simulink model "ACC_LQR_Gov_STALE"  (R2024a)
settings: Solver=FixedStepAuto  StartTime=0  StopTime=100  FixedStep=.05  RelTol=1e-3
undefined symbols (not defined in the file or in its folder): acc_max, acc_max_tight, Defined, driver_set_speed, Ego, jerk_max, k_I, k_vh, Lane, m, matlabshared, simStepSize, tau_lpf, User, v_dot_max
libraries: roadrunnerscenario x5, drivingscenarioandsensors x1, autolibshared x1
settings Model: PacingRate=10  Creator=darkh  LastModifiedBy=darkh
settings DataIOCC: ReturnWorkspaceOutputsName=sltest_internal_rrSimulationOutputVariable
settings OptimizationCC: ZeroExternalMemoryAtStartup=off  ZeroInternalMemoryAtStartup=off
settings DebuggingCC: AlgebraicLoopMsg=none
settings RTWCC: Description=Generate an RTMaps component embedding the model  SystemTargetFile=rtmaps.tlc  TemplateMakefile=rtmaps_default_tmf  PostCodeGenCommand=rtmaps_post_code_generation(buildInfo)  RetainRTWFile=on  TargetLang=C++  GPUComputeCapability=3.5
settings STFCustomTargetCC: TargetLangStandard=C++11 (ISO)  ModelReferenceCompliant=off  ConcurrentExecutionCompliant=on  CombineOutputUpdateFcns=on  CodeInterfacePackaging=C++ class  CPPClassGenCompliant=on  GRTInterface=off  UseToolchainInfoCompliant=off  SystemTargetFile=rtmaps.tlc
settings GRTTargetCC: TargetLangStandard=C++11 (ISO)  ModelReferenceCompliant=off  ParMdlRefBuildCompliant=off  CompOptLevelCompliant=off  MatFileLogging=off  CodeInterfacePackaging=C++ class  UseToolchainInfoCompliant=off
settings ConfigComp: CovSaveName=sltest_covdata  CovMetricSettings=dcmwe  CovEnableCumulative=off  CovSaveSingleToWorkspaceVar=on  CovSaveOutputData=off

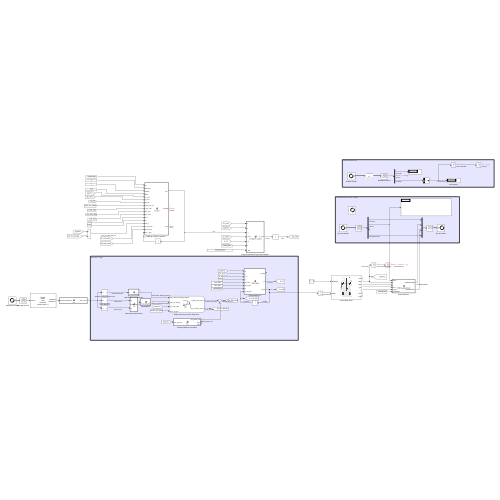
[thumbnail: Simulink's stored preview of the top-level diagram]
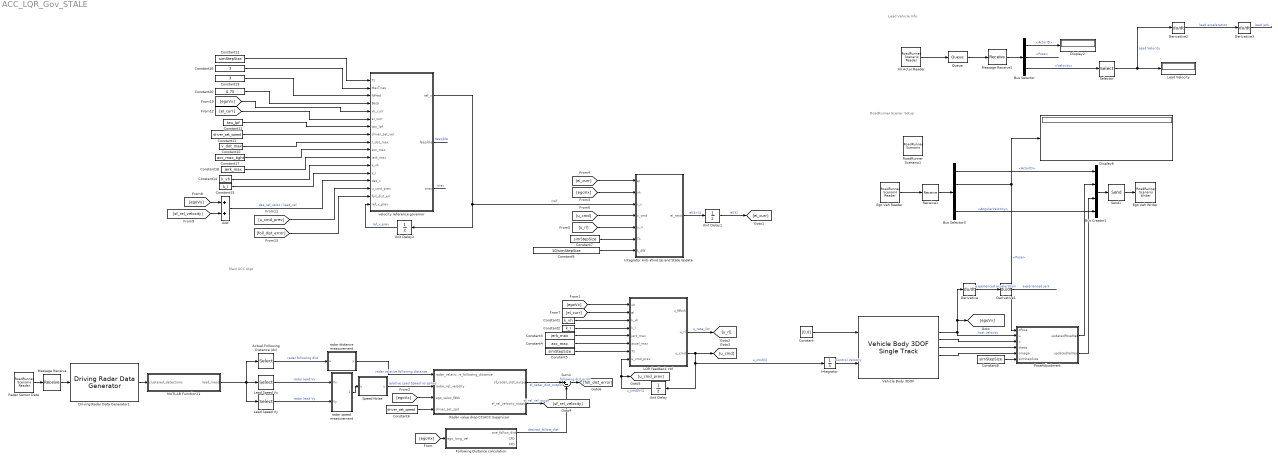
== system ACC_LQR_Gov_STALE ==
  note: RoadRunner Scenar. Setup
  note: Lead Vehicle Info.
  note: Main ACC Algo
  Actual Following Distance (dx) : Selector  InputPortWidth=6  IndexOptions=Index vector (dialog)  Indices=[1]  OutputSizes=1
  Add : Sum
  All Actor Reader : roadrunnerscenario/RoadRunner Scenario Reader  TopicCategory=Actor  ActorCategory=All Types  ActionType=Path Following  EventType=User-Defined  TopicType=Actor Pose  VehicleType=Vehicle Specifications  UserDefinedAction=Action1  UserDefinedEvent=Event1  Filter=None  SensorTopic=Target Poses  LaneBoundaryOutputTopic=Ego-Lane  SensorID=1  SampleTime=simStepSize
  Bus Creator1 : BusCreator  Inputs=4  OutDataTypeStr=Bus: BusActorRuntime  NonVirtualBus=on
      settings: InheritFromInputs=off
  Bus Selector : BusSelector  OutputSignals=ActorID,Pose,Velocity
  Bus Selector3 : BusSelector  OutputSignals=ActorID,Pose,Velocity,AngularVelocity
  Constant : Constant  Value=[0,0]
  Constant1 : Constant  Value=k_vh
  Constant10 : Constant  Value=v_dot_max
  Constant11 : Constant  Value=driver_set_speed
  Constant{5,7..8,12} (4 alike) : Constant  Value=simStepSize
  Constant13 : Constant  Value=tau_lpf
  Constant14 : Constant  Value=k_vh
  Constant15 : Constant  Value=k_I
  Constant16 : Constant  Value=3
  Constant17 : Constant  Value=acc_max_tight
  Constant18 : Constant  Value=jerk_max
  Constant19 : Constant  Value=3
  Constant2 : Constant  Value=k_I
  Constant20 : Constant  Value=0.75
  Constant3 : Constant  Value=jerk_max
  Constant4 : Constant  Value=acc_max
  Constant6 : Constant  Value=driver_set_speed
  Constant9 : Constant  Value=10/simStepSize
  Derivative{,1..3} (4 alike) : Derivative
  Display2 : Display
  Display6 : Display
  Driving Radar Data Generator1 : drivingscenarioandsensors/Driving Radar Data Generator  SensorIndex=1  UpdateRate=20  MountingLocation=[ 3.4, 0, 0.2 ]  MountingAngles=[0 0 0]  HasElevation=off  HasRangeRate=on  HasNoise=off  HasFalseAlarms=off  HasOcclusion=on  MaxNumReportsSource=Property  MaxNumReports=50  TargetReportFormat=Clustered detections  DetectionCoordinates=Body  TrackCoordinates=Body  BusNameSource=Auto  BusName=BusDrivingRadarDataGenerator  AzimuthResolution=4  ElevationResolution=5  RangeResolution=2.5  RangeRateResolution=0.5  AzimuthBiasFraction=0.1  ElevationBiasFraction=0.1  RangeBiasFraction=0.05  RangeRateBiasFraction=0.05  FieldOfView=[ 20, 5 ]  RangeLimits=[ 0, 150 ]  RangeRateLimits=[ -100, 100 ]  DetectionProbability=0.9  FalseAlarmRate=1e-06  ReferenceRange=100  ReferenceRCS=0  CenterFrequency=77e9  FilterInitializationFcn=initcvekf  ConfirmationThreshold=[2 3]  DeletionThreshold=[5 5]  InitialSeedSource=Repeatable  InitialSeed=0  UsedSeed=matlabshared.tracking.internal.SimulinkUtilities.seedManager(gcb)  ProfilesSource=From Scenario Reader block  ProfilesParameters=driving.internal.ActorProfilesRadarParameters  ProfilesExpression=struct('ClassID',0,'Length',4.7,'Width',1.8,'Height',1.4,'OriginOffset',[-1.35 0 0],'RCSPattern',[10 10;10 10],'RCSAzimuthAngles',[-180 180],'RCSElevationAngles',[-90 90])
  Ego Veh Reader : roadrunnerscenario/RoadRunner Scenario Reader  TopicCategory=Actor  ActorCategory=All Types  ActionType=Path Following  EventType=User-Defined  TopicType=Actor Pose  VehicleType=Vehicle Specifications  UserDefinedAction=Action1  UserDefinedEvent=Event1  Filter=Self  SensorTopic=Target Poses  LaneBoundaryOutputTopic=Ego-Lane  SensorID=1  SampleTime=simStepSize
  Ego Veh Writer : roadrunnerscenario/RoadRunner Scenario Writer  TopicCategory=Actor  ActorCategory=All Types  EventType=Action Complete  UserDefinedEvent=Event1  VehicleType=Vehicle Pose  TopicType=Actor Pose
  Following Distance calculation : MATLAB Function  TreatAsAtomicUnit=on
  Integrator : Integrator
  Integrator Anti-Wind Up and State Update : MATLAB Function  TreatAsAtomicUnit=on
  LQR feedback ctrl : MATLAB Function  TreatAsAtomicUnit=on
  Lead Speed Vx : Selector  InputPortWidth=6  IndexOptions=Index vector (dialog)  Indices=4  OutputSizes=1
  Lead Speed Vy : Selector  InputPortWidth=6  IndexOptions=Index vector (dialog)  Indices=5  OutputSizes=1
  Lead Velocity : Display
  MATLAB Function11 : MATLAB Function  TreatAsAtomicUnit=on
  Message Receive : Receive  InputPortMessageModes=m  UseInternalQueue=off
  Message Receive1 : Receive  InputPortMessageModes=m
  PoseAdjustment : MATLAB Function  TreatAsAtomicUnit=on
  Queue : Queue  InputPortMessageModes=m  OutputPortMessageModes=m  OverwriteOldest=on  Capacity=16  QueueType=LIFO
  Radar Sensor Data : roadrunnerscenario/RoadRunner Scenario Reader  TopicCategory=Sensor  ActorCategory=All Types  ActionType=Path Following  EventType=User-Defined  TopicType=Actor Specifications  VehicleType=Vehicle Specifications  UserDefinedAction=Action1  UserDefinedEvent=Event1  Filter=Self  SensorTopic=Target Poses  LaneBoundaryOutputTopic=Ego-Lane  SensorID=1  SampleTime=simStepSize
  Radar value drop CC/ACC Supervisor : Stateflow chart  TreatAsAtomicUnit=on
  Receive1 : Receive  InputPortMessageModes=m  UseInternalQueue=off  QueueOverwriting=on  QueueLength=1  QueueType=LIFO
  RoadRunner Scenario1 : roadrunnerscenario/RoadRunner Scenario  UserDefinedActions={}  UserDefinedEvents={}
  Selector : Selector  InputPortWidth=3  IndexOptions=Index vector (dialog)  Indices=[2]  OutputSizes=1
  Send1 : Send  OutputPortMessageModes=m
  Speed Noise : MATLAB Function  TreatAsAtomicUnit=on
  Sum4 : Sum  Inputs=|+-
  Unit Delay : UnitDelay  SampleTime=-1  HasFrameUpgradeWarning=on
  Unit Delay1 : UnitDelay  SampleTime=-1  HasFrameUpgradeWarning=on
  Unit Delay2 : UnitDelay  SampleTime=-1  HasFrameUpgradeWarning=on
  "Vehicle Body 3DOF " : autolibshared/Vehicle Body 3DOF Single Track  trackMode=Dual  inputMode=External longitudinal velocity  frontSteerMode=on  rearSteerMode=off  windMode=off  muMode=off  extFMode=off  extMMode=off  htchFMode=off  htchMMode=off  extXo=off  extpsio=off  extxdoto=off  extro=off  extYo=off  extTamb=off  extydoto=off  aMode=2  NF=2  NR=2  m=m  a=1.5569  b=1.5371  h=0.18903  dh=1  hh=0.2  X_o=0  xdot_o=0  CalphaMode=off  sigmaMode=on  d=0  hl=0  w=[1.4,1.4]  Cy_f=40000  Cy_r=40000  sigma_f=.1  sigma_r=.1  alpha_f_brk=[-.1 .1]  Cy_f_data=[-9e3 9e3]  alpha_r_brk=[-.1 .1]  Cy_r_data=[-9e3 9e3]  Y_o=0  ydot_o=0  Izz=2066  psi_o=0  r_o=0  Af=2.73  Cd=.30356  Cl=.1  Cpm=.1  beta_w=[0 0.01:0.01:0.3]  Cs=[0 0.01:0.01:0.3]  Cym=[0 1e-6:0.01:0.3]  Pabs=101325  Tair=273  g=9.81  mu=1  xdot_tol=.01  Fznom=5000  Fxtire_sat=7e4  Fytire_sat=7e4  longOff=0  latOff=0  vertOff=0  wrapAng=off
  radar distance measurement : MATLAB Function  TreatAsAtomicUnit=on
  radar speed measurement : MATLAB Function  TreatAsAtomicUnit=on
  velocity reference governor : MATLAB Function  TreatAsAtomicUnit=on  SystemSampleTime=simStepSize
  wires:
  Bus Selector3/4 -> Bus Creator1/4  "<AngularVelocity>"
  Bus Creator1/1 -> Send1/1
  Bus Selector3/1 -> Bus Creator1/1  "<ActorID>"
  Receive1/1 -> Bus Selector3/1
  Send1/1 -> Ego Veh Writer/1
  Ego Veh Reader/1 -> Receive1/1
  Bus Selector3/2 -> Display6/1, PoseAdjustment/1(cPose)  "<Pose>"
  PoseAdjustment/1(updatedPoseMat) -> Bus Creator1/2
  "Vehicle Body 3DOF "/2 -> Derivative/1, [egoVx], PoseAdjustment/2(u)  "host velocity"
  Radar Sensor Data/1 -> Message Receive/1
  Message Receive/1 -> Driving Radar Data Generator1/1
  Driving Radar Data Generator1/1 -> MATLAB Function11/1(clustered_detections)
  PoseAdjustment/2(updatedVelVec) -> Bus Creator1/3
  Integrator/1 -> "Vehicle Body 3DOF "/2  "Control Velocity"
  Constant/1 -> "Vehicle Body 3DOF "/1
  Speed Noise/1(y) -> Radar value drop CC/ACC Supervisor/2(radar_rel_velocity)  "relative Lead Speed no spikes"
  Lead Speed Vx/1 -> radar speed measurement/1(Vx)  "radar lead Vx"
  [egoVx] -> Following Distance calculation/1(ego_long_vel)
  MATLAB Function11/1(lead_meas) -> Lead Speed Vy/1, Actual Following Distance (dx)/1, Lead Speed Vx/1
  radar distance measurement/1(y) -> Radar value drop CC/ACC Supervisor/1(radar_relative_following_distance)  "radar relative following distance"
  Lead Speed Vy/1 -> radar speed measurement/2(Vy)  "radar lead Vy"
  radar speed measurement/1(LeadSpeed) -> Speed Noise/1(u)
  Actual Following Distance (dx)/1 -> radar distance measurement/1(u)  "radar following dist"
  Derivative/1 -> Derivative1/1  "experienced acceleration"
  Derivative1/1 -> ?  "experienced jerk"
  Constant6/1 -> Radar value drop CC/ACC Supervisor/4(driver_set_spd)
  Constant8/1 -> PoseAdjustment/6(simStepSize)
  "Vehicle Body 3DOF "/4 -> PoseAdjustment/4(theta)
  "Vehicle Body 3DOF "/5 -> PoseAdjustment/5(omega)
  "Vehicle Body 3DOF "/3 -> PoseAdjustment/3(v)
  All Actor Reader/1 -> Queue/1
  Queue/1 -> Message Receive1/1
  Message Receive1/1 -> Bus Selector/1
  Bus Selector/1 -> Display2/1  "<ActorID>"
  Bus Selector/2 -> ?  "<Pose>"
  Bus Selector/3 -> Selector/1  "<Velocity>"
  Selector/1 -> Derivative2/1, Lead Velocity/1  "Lead Velocity"
  Derivative2/1 -> Derivative3/1  "lead acceleration"
  Derivative3/1 -> ?  "lead jerk"
  Sum4/1 -> [foll_dist_error]  "following dist error"
  [egoVx] -> LQR feedback ctrl/1(vh)
  Constant1/1 -> LQR feedback ctrl/3(k_vh)
  Constant2/1 -> LQR feedback ctrl/4(k_I)
  Constant3/1 -> LQR feedback ctrl/5(jerk_max)
  Constant4/1 -> LQR feedback ctrl/6(accel_max)
  Constant5/1 -> LQR feedback ctrl/7(Ts)
  LQR feedback ctrl/3(u_cmd) -> Integrator/1, Unit Delay/1, [u_cmd]  "u_cmd[k]"
  Unit Delay/1 -> LQR feedback ctrl/8(u_cmd_prev), [u_cmd_prev]  "u_cmd[k-1]"
  [egoVx] -> Radar value drop CC/ACC Supervisor/3(ego_veloc_fdbk)
  Following Distance calculation/1(ave_follow_dist) -> Sum4/2  "desired_follow_dist"
  Radar value drop CC/ACC Supervisor/1(sf_radar_dist_output) -> Sum4/1  "sf_radar_dist_output"
  Integrator Anti-Wind Up and State Update/1(eI_next) -> Unit Delay1/1  "eI[k+1]"
  Constant7/1 -> Integrator Anti-Wind Up and State Update/6(Ts)
  [egoVx] -> Integrator Anti-Wind Up and State Update/2(vh)
  Unit Delay1/1 -> [eI_curr]  "eI[k]"
  [eI_curr] -> Integrator Anti-Wind Up and State Update/1(eI)
  LQR feedback ctrl/2(u_rl) -> [u_rl]  "u_rate_lim"
  [u_rl] -> Integrator Anti-Wind Up and State Update/5(u_rl)
  [u_cmd] -> Integrator Anti-Wind Up and State Update/4(u_cmd)
  [eI_curr] -> LQR feedback ctrl/2(eI)
  velocity reference governor/1(ref_v) -> Unit Delay2/1, Integrator Anti-Wind Up and State Update/3(r_v)  "vref"
  Constant9/1 -> Integrator Anti-Wind Up and State Update/7(k_AW)
  Radar value drop CC/ACC Supervisor/2(sf_rel_velocity_output) -> [sf_rel_velocity]  "sf_rel_vel_outpt"
  [egoVx] -> Add/1
  [sf_rel_velocity] -> Add/2
  Add/1 -> velocity reference governor/14(des_v)  "des_ref_veloc / lead_vel"
  Unit Delay2/1 -> velocity reference governor/17(ref_v_prev)  "ref_v_prev"
  Constant12/1 -> velocity reference governor/1(Ts)
  Constant13/1 -> velocity reference governor/7(tau_lpf)
  Constant14/1 -> velocity reference governor/12(k_vh)
  Constant15/1 -> velocity reference governor/13(k_I)
  Constant10/1 -> velocity reference governor/9(r_dot_max)
  Constant11/1 -> velocity reference governor/8(driver_set_vel)
  [egoVx] -> velocity reference governor/5(vh_curr)
  [u_cmd_prev] -> velocity reference governor/15(u_cmd_prev)
  [eI_curr] -> velocity reference governor/6(eI_curr)
  Constant16/1 -> velocity reference governor/2(MaxTries)
  [foll_dist_error] -> velocity reference governor/16(foll_dist_err)
  Constant17/1 -> velocity reference governor/10(acc_max)
  Constant18/1 -> velocity reference governor/11(jerk_max)
  Constant19/1 -> velocity reference governor/3(NPred)
  Constant20/1 -> velocity reference governor/4(Beta)
  velocity reference governor/2(feasible) -> ?  "feasible"
  velocity reference governor/3(tries) -> ?  "tries"

== matlab function ACC_LQR_Gov_STALE/PoseAdjustment ==
  data: cPose input; u input; updatedPoseMat output; v input; theta input; omega input; updatedVelVec output; simStepSize input
function [updatedPoseMat, updatedVelVec] = RRPoseAdjustment(cPose, u, v, theta, omega, simStepSize)
    thetad = theta + omega*simStepSize;
    xd = (u*cos(theta) - v*sin(theta))*simStepSize;
    yd = (u*sin(theta) + v*cos(theta))*simStepSize;
    pose_mat = [cos(-thetad) -sin(-thetad) 0 (yd+cPose(1,4)); sin(-thetad) cos(-thetad) 0 (xd+cPose(2,4)); 0 0 1 0; 0 0 0 1];
    updatedPoseMat = pose_mat;
    updatedVelVec = [u*sin(theta) + v*cos(theta), u*cos(theta) - v*sin(theta), 0];
    return;
end

== matlab function ACC_LQR_Gov_STALE/radar distance measurement ==
  data: u input; y output
function y = removeSpikes(u)

    persistent buffer;
    persistent bufferIndex;
    threshold = 2;
    % windowSize = 15;
    windowSize = 5;
    
    if isempty(buffer)
        buffer = zeros(1, windowSize);
        bufferIndex = 1;
    end
    
    % Update buffer with new value
    buffer(bufferIndex) = u;
    bufferIndex = mod(bufferIndex, windowSize) + 1;
    
    % Calculate the median of the buffer
    medVal = median(buffer);
    
    % Detect and remove spikes
    if abs(u - medVal) > threshold
        y = medVal; % Replace spike with the median value
    else
        y = u; % Keep the original value if it's not a spike
    end
end

== matlab function ACC_LQR_Gov_STALE/radar speed measurement ==
  data: Vx input; LeadSpeed output; Vy input
function LeadSpeed = fcn(Vx, Vy)

if Vx == 0 && Vy == 0 
    Vx = 0.01;
    Vy = 0.01;
elseif Vy == 0
    Vy = 0.01;
elseif Vx == 0
    Vx = 0.01;
end

if Vx <= 0
    LeadSpeed = -sqrt(Vx^2 + Vy^2);
else
    LeadSpeed = sqrt(Vx^2 + Vy^2);
end

== matlab function ACC_LQR_Gov_STALE/Speed Noise ==
  settings: updateMethod=DISCRETE
  data: u input; y output
function y = removeSpikes(u)
    % removeSpikes - Removes spikes from a scalar signal based on a threshold
    %
    % Inputs:
    %    u - The input signal (scalar)
    %    threshold - The threshold value to detect spikes
    %    windowSize - The size of the window for calculating the median
    %
    % Outputs:
    %    y - The filtered signal with spikes removed

    % Declare persistent variables to store past values
    persistent buffer;
    persistent bufferIndex;
    threshold = 2;
    % windowSize = 15;
    windowSize = 5;

    
    if isempty(buffer)
        buffer = zeros(1, windowSize);
        bufferIndex = 1;
    end
    
    % Update buffer with new value
    buffer(bufferIndex) = u;
    bufferIndex = mod(bufferIndex, windowSize) + 1;
    
    % Calculate the median of the buffer
    medVal = median(buffer);
    
    % Detect and remove spikes
    if abs(u - medVal) > threshold
        y = medVal; % Replace spike with the median value
    else
        y = u; % Keep the original value if it's not a spike
    end
end

== matlab function ACC_LQR_Gov_STALE/MATLAB Function11 ==
  data: clustered_detections input Bus: BusRadar; lead_meas output double
function lead_meas = fcn(clustered_detections)

lead_det = clustered_detections.Detections(1);
lead_meas = lead_det.Measurement;

% relative_dist = sqrt(lead_det.Measurement(1)^2 + lead_det.Measurement(2)^2); % rel_dist = sqrt(x^2+y^2)
% relative_speed = sqrt(lead_det.Measurement(4)^2 + lead_det.Measurement(5)^2);
end

== matlab function ACC_LQR_Gov_STALE/Following Distance calculation ==
  settings: updateMethod=DISCRETE
  data: ego_long_vel input; ave_follow_dist output; CFD output; FFD output
% Function to determine the closest (CFD) and furthest follow distance (FFD) for the
% ego vehicle relative to the lead vehicle given the ego vehicle's current
% velocity

% This function outputs the middle distance value between the CFD and FFD
% and those values respectively as well

function [ave_follow_dist, CFD, FFD] = fcn(ego_long_vel)
    persistent dist_history window_size smoothing_weights
    
    % Initialize (first call only)
    if isempty(dist_history)
        window_size = 5;  % Number of past samples
        dist_history = zeros(1, window_size);
        
        % Define and normalize weights (e.g., linear decay)
        smoothing_weights = linspace(1, 0.5, window_size);  % Weights from 1.0 to 0.5
        smoothing_weights = smoothing_weights / sum(smoothing_weights);  % Normalize
    end
    ego_long_vel_mph = ego_long_vel*2.23694;
    
    if ego_long_vel_mph > 0 && ego_long_vel_mph < 20
        CFD = 2.8*ego_long_vel_mph^0.45+8;
        FFD = 100-0.2*(20-ego_long_vel_mph)^2;
    elseif ego_long_vel_mph <= 0
        CFD = 8;
        FFD = 100-0.2*(20)^2;
    else
        CFD = 2.8*ego_long_vel_mph^0.45+8;
        FFD = 100;
    end
    AveFollowDist_Gain = 3; % As this gets larger, desired distance is set closer to lead vehicle


    % --- Update history buffer ---
    dist_history = [ ((AveFollowDist_Gain-1)*CFD + FFD)/AveFollowDist_Gain , dist_history(1:end-1)];  % FIFO

    % --- Smoothed average (weighted, normalized) ---
    smoothed_ave_dist = sum(dist_history .* smoothing_weights);
    
    % --- Clamp to CFD/FFD bounds ---
    ave_follow_dist = min(max(smoothed_ave_dist, CFD), FFD);
end

== matlab function ACC_LQR_Gov_STALE/Integrator Anti-Wind Up and State Update ==
  data: eI input; eI_next output; vh input; r_v input; u_cmd input; u_rl input; Ts input; k_AW input
function eI_next  = integrator_update(eI, vh, r_v, u_cmd, u_rl, Ts, k_AW)

% This function block takes in the current integrator state eI[k], as well
% as u_cmd and u_rl to perform Anti-Wind up with back calculation on the
% integrator due to control signal saturation; k_AW is integrator back calculation gain
eI = eI + k_AW*(u_cmd - u_rl)*Ts; % Bleeding integrator state at current timestep before updating

% current vehicle speed error e_vh[k] = r_v[k] - vh[k] is used to update the
% integrator state for next time step eI[k+1] = eI[k] + e_vh[k] * Ts
e_vh = r_v - vh;
eI_next = eI + e_vh*Ts;

== matlab function ACC_LQR_Gov_STALE/LQR feedback ctrl ==
  data: vh input; u_fdbck output; eI input; k_vh input; k_I input; jerk_max input; accel_max input; Ts input; u_cmd_prev input; u_rl output; u_cmd output
function [u_fdbck, u_rl, u_cmd] = LQR_fdbck(vh, eI, k_vh, k_I, jerk_max, accel_max, Ts, u_cmd_prev)
% 
% This takes in the current host velocity and integrator states, LQR gains for velocity and integrator states, as well as jerk and acceleration limits to generate final control signal

% u_fdbck is the feedback control acceleration from the control law u = -k_x * x - k_I * eI given the LQR feedback gains generated
u_fdbck = - k_vh*vh - k_I*eI; % raw LQR control signal

u_rl = min(max(u_fdbck, u_cmd_prev - jerk_max*Ts), u_cmd_prev + jerk_max*Ts); % applying jerk rate limits; u_rl = clip(u_fdbck, u_prev - du_max*Ts, u_prev + du_max*Ts)
u_cmd = min(max(u_rl, -accel_max), accel_max); % applied acceleration limits; u_cmd = clip(u_rl, u_min, u_max)

== stateflow chart ACC_LQR_Gov_STALE/Radar value drop CC//ACC Supervisor ==
  state Radar_State_Lead_Veh_Present_and_Detected
    sf_radar_dist_output = radar_relative_following_distance;
    sf_rel_velocity_output = radar_rel_velocity;
  state Output_Spoof_To_Keep_Moving
    sf_radar_dist_output = 150;
    % sf_radar_dist_output = smooth_switch(sf_radar_dist_output, 150, 0.05, 2);
    set_spd_err = driver_set_spd - ego_veloc_fdbk;
    sf_rel_velocity_output = set_spd_err;
    % sf_rel_velocity_output = smooth_switch(sf_rel_velocity_output, set_spd_err, 0.05, 5);
  (default) -> Radar_State_Lead_Veh_Present_and_Detected : {sf_radar_dist_output = radar_relative_following_distance;
      | sf_rel_velocity_output = radar_rel_velocity;}
  Radar_State_Lead_Veh_Present_and_Detected -> Output_Spoof_To_Keep_Moving : [radar_relative_following_distance == 0 && radar_rel_velocity < 0.9]
  Output_Spoof_To_Keep_Moving -> Radar_State_Lead_Veh_Present_and_Detected : [radar_relative_following_distance > 0]
  data: prev_val function_input; curr_val function_input; dt function_input; tau function_input; filtered_val function_output; radar_relative_following_distance input; sf_radar_dist_output output; radar_rel_velocity input; ego_veloc_fdbk input; sf_rel_velocity_output output; driver_set_spd input; set_spd_err local
  function filtered_val = smooth_switch(prev_val, curr_val, dt, tau):
    | function filtered_val = smooth_switch(prev_val, curr_val, dt, tau)
    | % Smooth transition from prev_val toward curr_val
    | % dt  = sample time [s]; equal to system sample time of 0.05s currently
    | % tau = time constant [s] (0.3–1.0 typical)
    | 
    | if isempty(prev_val)
    |     prev_val = 0;
    | end
    | 
    | alpha = exp(-dt/tau);
    | filtered_val = alpha*prev_val + (1-alpha)*curr_val;
    | end

== matlab function ACC_LQR_Gov_STALE/velocity reference governor ==
  data: Ts input; MaxTries input; NPred input; Beta input; vh_curr input; eI_curr input; tau_lpf input; driver_set_vel input; r_dot_max input; acc_max input; jerk_max input; k_vh input; ref_v output; k_I input; des_v input; u_cmd_prev input; foll_dist_err input; ref_v_prev input; feasible output; tries output
function [ref_v, feasible, tries] = ref_gov(Ts, MaxTries, NPred, Beta, vh_curr, eI_curr, tau_lpf, driver_set_vel, r_dot_max, acc_max, jerk_max, k_vh, k_I, des_v, u_cmd_prev, foll_dist_err, ref_v_prev)
% generates the reference velocity signal for the integrator to track,
% generates velocity by predicting closed loop performance over a moving
% window of ~N=3 timesteps; Generated velocity reference is kept within
% bounds of jerk and applied acceleration limits; If prediction loop is not
% within bounds, then reference change is tightened and re-predicted up to M times, if
% successful the control determined is applied, otherwise the previous
% safest control signal is applied

% Inputs:
%  r_dot_max : slew rate for reference velocity signal, how much change in velocity is allowed per unit of time given a change in desired reference; m/s^2
%  MaxTries : maximum attempts at determining a reference velocity signal until the previous output is just used again

% Outputs:
%  r_next   : next admissible reference [m/s]
%  feasible : 1 if proposed step accepted without backoff
%  tries    : number of backoff steps used

% Reconstructing the closed loop augmented with integrator system to
% predict system's response to proposed reference velocities
m = 2630.84; % kg; mass of LYRIQ
Cw = 0.30356; % LYRIQ wind resistance coeff
Aw = 2.73; % m^2 windward area of the LYRIQ
rho = 1.206; % kg/m^3 air density
aero_const = Cw*Aw*rho/2;
vh_nom = 30; % for when keeping the d7rag term constant
Ac = -aero_const*vh_nom/m; % Single state plant x = vh
Bc = 1;
Ad = 1 + Ac.*Ts; % Using Euler discretization to obtain the discrete time matrices from the continuous time system
Bd = Bc.*Ts;
Acl = [Ad-Bd*k_vh, -Bd*k_I; -Ts, 1.0]; % Closed loop system matrix
Br = [0.0; Ts]; % matrix for including reference velocity term in the integrator

% persistent variable for the low pass filter on the desired velocity
persistent r_lpf
if isempty(r_lpf)
    r_lpf = ref_v_prev;
end
alpha = Ts/(tau_lpf + Ts);
r_lpf = r_lpf + alpha*(des_v - r_lpf); % Computing the low pass filtered value from desired reference velocity
r_try = min(max(r_lpf, ref_v_prev - r_dot_max*Ts), ref_v_prev + r_dot_max*Ts); % clipping low pass filtered reference velocity to follow desired change in velocity bounds; slew rate
r_try = min(max(r_try, 0.0), driver_set_vel); % Clipping reference velocity between [0, driver set limit]

step = r_try - ref_v_prev; % velocity step size between current ref velocity and previous output

% initialization of variables to hold prediction states over for loops
x_init = [vh_curr; eI_curr];
u_init = u_cmd_prev;
feasible = 0;
tries = 0;

vlead_hat = des_v; % the lead vehicle's velocity is effectively the same as the desired velocity

for attempt = 0:MaxTries
    % reset predicted states each attempt
    x_i = x_init;
    u_i = u_init;
    derr_i = foll_dist_err;  % carry distance error forward for checks

    ok = true;

    for i = 1:NPred
        % Propagate augmented closed loop (2x2) with constant r_try
        x_i = Acl * x_i + Br * r_try;
        vp   = x_i(1);
        eIp  = x_i(2);
        % Reconstruct predicted accel (LQR)
        u = -(k_vh * vp + k_I * eIp);

        % % 3) (Optional) mirror jerk clamp inside prediction
        % if ~isempty(gov.DuStepPred)
        %     u = clip(u, u_i - gov.DuStepPred, u_i + gov.DuStepPred);
        % end

        % Accel bound (tightened)
        u = min(max(u, -acc_max), acc_max);

        % Checking Speed bound (tight with small margin)
        if (vp < 0.0) || (vp > driver_set_vel + 2.0) % 2.0 m/s is margin
            ok = false;
            break;
        end

        % Checking Jerk bound; if either bounds are violated, the prediction loop is exited
        if abs(u - u_i) > (jerk_max*Ts + 1e-12)
            ok = false;
            break;
        end

        % Distance-error check (constant-distance policy); Propagate derr one step: derr_{k+1} = derr_k + Ts*(v_lead - v)
        derr_i = derr_i + Ts*(vlead_hat - vp);

        % Guard: enforce derr >= DerrMin + margin
        if derr_i < (0.0 + 2.0) % 0.0 is the DerrMin and 2.0 is the margin [m]
            ok = false;
            break;
        end  

        % advance
        u_i = u;
    end

    if ok
        feasible = 1 * (attempt == 0);
        ref_v = r_try;
        tries = attempt;
        return;
    else
        % backoff step toward last safe r_prev
        step = Beta * step; % Shortening the step size by beta
        r_try = ref_v_prev + step; % newer shorter step size
        r_try = min(max(r_try, 0.0), driver_set_vel);  % keep inside band
    end
end

% If we get here, hold last reference (safe fallback)
ref_v = ref_v_prev;
% ref_v = r_try; % For when testing without the prediction loop and want to output the raw r_try
feasible = 0;
tries = MaxTries;
